simulink model "simulink_sim_V1"  (R2017a)
settings: Solver=FixedStepDiscrete  StartTime=0  StopTime=7  FixedStep=Ts  RelTol=1e-3  EnableMultiTasking=on
values from neighbouring files (symbols this model uses):
  Ts = 0.025    [ACADO_simulink.m]
  Xref = [0 0 0 0]    [ACADO_simulink.m]
undefined symbols (not defined in the file or in its folder): data, init, sigbuilder_block
settings Model: Creator=hirsch  LastModifiedBy=alvin
settings DataIOCC: LimitDataPoints=on  SaveFormat=Array  SignalLoggingSaveFormat=ModelDataLogs
settings OptimizationCC: ExpressionDepthLimit=2147483647  LifeSpan=inf
settings DebuggingCC: SolverPrmCheckMsg=warning  FcnCallInpInsideContextMsg=warning  StateNameClashWarn=warning  SFUnexpectedBacktrackingDiag=warning  SFNoUnconditionalDefaultTransitionDiag=warning  SFExecutionAtInitializationDiag=none
settings HardwareCC: ProdBitPerPointer=32  ProdBitPerSizeT=32  ProdBitPerPtrDiffT=32  ProdLargestAtomicFloat=None  ProdIntDivRoundTo=Undefined  ProdEndianess=Unspecified  ProdWordSize=32  ProdHWDeviceType=32-bit Generic
settings ModelReferenceCC: PropagateSignalLabelsOutOfModel=off
settings GRTTargetCC: TargetLangStandard=C89/C90 (ANSI)  GeneratePreprocessorConditionals=Disable all  CombineOutputUpdateFcns=off  GRTInterface=on
settings ConfigComp: CovMetricSettings=dw  CovHtmlReporting=on  CovSaveCumulativeToWorkspaceVar=on  CovSaveSingleToWorkspaceVar=on  CovExternalEMLEnable=off  CovSFcnEnable=off

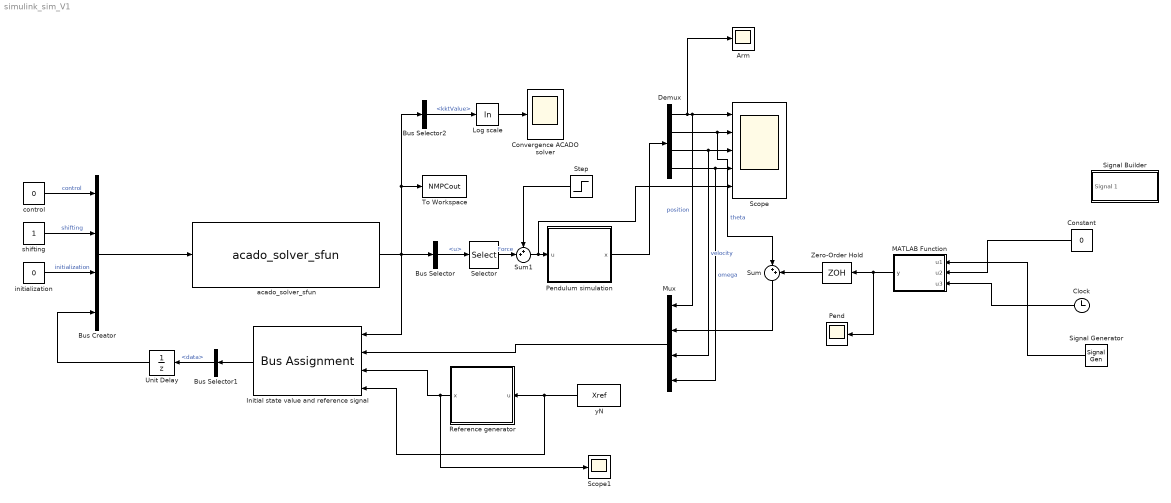
== system simulink_sim_V1 ==
  Arm : Scope
  Bus Creator : BusCreator  Inputs=4  OutDataTypeStr=Bus: ACADOinput
  Bus Selector : BusSelector  OutputSignals=data.u
  Bus Selector1 : BusSelector  OutputSignals=data
  Bus Selector2 : BusSelector  OutputSignals=kktValue
  Clock : Clock
  Constant : Constant  Value=0
  Convergence ACADO solver : Scope
  Demux : Demux
  Initial state value and reference signal : BusAssignment  AssignedSignals=data.x0,data.y,data.yN
  Log scale : Math  Operator=log  SaturateOnIntegerOverflow=on
  MATLAB Function : MATLAB Function  TreatAsAtomicUnit=on
  Mux : Mux
  Pend : Scope
  Pendulum simulation : Subsystem
      mask help: Simple system simulation.
      mask init:
      | % initialize state values
      mask Display: disp('System');
  Reference generator : Subsystem
      mask help: Simple system simulation.
      mask init:
      | % initialize state values
      mask Display: disp('System');
  Scope : Scope  NumInputPorts=5
  Scope1 : Scope
  Selector : Selector  InputPortWidth=80  IndexOptions=Starting index (dialog)  Indices=[1]  OutputSizes=1
  Signal Generator : SignalGenerator  Amplitude=0.1  Frequency=10  Units=rad/sec
  Signal Builder : Subsystem  Tag=STV Subsys  LoadFcn=sigbuilder_block('load');  StartFcn=sigbuilder_block('start');  StopFcn=sigbuilder_block('stop');  ClipboardFcn=sigbuilder_block('clipboard');  mask(Sigbuilder block){tuvar=[0:10]}
      mask help: Simulink:masks:SigbuilderBlock_MD
      mask init:
      | if ~strcmp(get_param(bdroot(gcbh),'SimulationStatus'),'stopped') tuvar = sigbuilder_block('maskInit'); end
      settings: CopyFcn=sigbuilder_block('copy');  DeleteFcn=sigbuilder_block('delete');  ModelCloseFcn=sigbuilder_block('modelClose');  PreSaveFcn=sigbuilder_block('preSave');  PauseFcn=sigbuilder_block('pause');  ContinueFcn=sigbuilder_block('continue');  NameChangeFcn=sigbuilder_block('namechange');  OpenFcn=sigbuilder_block('open',[94.5 0 580.5 448.5 ]);  CloseFcn=sigbuilder_block('close');
      mask Display: plot(0, 0, 100, 100,[2, 2, 32, 32, 2], [68, 8, 8, 68, 68],[32, 2], [38, 38], [32, 19, 2],[53, 60, 44], [32, 17, 17, 2],[16, 16, 31, 31]);txt = getActiveGroup(gcbh);text(2, 100, txt,'verticalAlignment', 'top');
  Step : Step  Time=4  After=0  SampleTime=0
  Sum : Sum  Inputs=|++
  Sum1 : Sum  Inputs=++|
  To Workspace : ToWorkspace  VariableName=NMPCout  SaveFormat=Timeseries  SampleTime=-1
  Unit Delay : UnitDelay  InitialCondition=init  SampleTime=Ts
  Zero-Order Hold : ZeroOrderHold  SampleTime=0.025
  acado_solver_sfun : S-Function  FunctionName=acado_solver_sfun  SFunctionDeploymentMode=off  EnableBusSupport=off  mask(Legacy Function){SFunctionSpec=acado_step(ACADOinput u1[1], ACADOoutput y1[1]), ShowSpec=on}
      mask prompts: ShowSpec "Display function specification"
      mask help:
      | This block allows you to call the legacy functions specified by the following Legacy Code Tool definition:
      | def.SFunctionName = 'acado_solver_sfun';
      | def.OutputFcnSpec = 'acado_step(ACADOinput u1[1], ACADOoutput y1[1])';
      | def.StartFcnSpec = 'acado_initialize( void )';
      | def.TerminateFcnSpec = 'acado_cleanup( void )';
      | def.HeaderFiles = {'acado_common.h', 'acado_solver_sfunction.h'};
      | def.SourceFiles = {'acado_solver.c', 'acado_integrator.c', 'acado_auxiliary_functions.c', 'acado_solver_sfunction.c', 'acado_qpoases_interface.cpp', 'qpoases/SRC/Bounds.cpp', 'qpoases/SRC/Constraints.cpp', 'qpoases/SRC/CyclingManager.cpp', 'qpoases/SRC/Indexlist.cpp', 'qpoases/SRC/MessageHandling.cpp', 'qpoases/SRC/QProblem.cpp', 'qpoases/SRC/QProblemB.cpp', 'qpoases/SRC/SubjectTo.cpp', 'qpoases/SRC/Utils.cpp', 'qpoases/SRC/EXTRAS/SolutionAnalysis.cpp'};
      | def.IncPaths = {'qpoases', 'qpoases/INCLUDE', 'qpoases/SRC'};
      | def.Options.language = 'C++';
      mask Help: <p>This block was generated automatically by the Legacy Code Tool. For detailed help on this tool, call<a href="matlab:legacy_code('help')"> legacy_code('help')</a>.</p>
      mask Callback ShowSpec:
      | if strcmp(get_param(gcbh, 'ShowSpec'), 'on')
      |   set_param(gcbh, 'MaskDisplay', sprintf('fprintf(''%s'');', get_param(gcbh, 'SFunctionSpec')));
      | else
      |   set_param(gcbh, 'MaskDisplay', sprintf('fprintf(''%s'');', get_param(gcbh, 'FunctionName')));
      | end
      mask Display: fprintf('acado_step(ACADOinput u1[1], ACADOoutput y1[1])');
  control : Constant  Value=0  OutDataTypeStr=int32
  initialization : Constant  Value=0  OutDataTypeStr=int32
  shifting : Constant  OutDataTypeStr=int32
  yN : Constant  Value=Xref  OutDataTypeStr=double
  wires:
  acado_solver_sfun/1 -> Bus Selector2/1, To Workspace/1, Initial state value and reference signal/1, Bus Selector/1
  Bus Selector/1 -> Selector/1  "<u>"
  shifting/1 -> Bus Creator/2  "shifting"
  control/1 -> Bus Creator/1  "control"
  initialization/1 -> Bus Creator/3  "initialization"
  Initial state value and reference signal/1 -> Bus Selector1/1
  Demux/1 -> Arm/1, Mux/1, Scope/1  "position"
  Demux/2 -> Sum/1, Scope/2  "theta"
  Demux/3 -> Mux/3, Scope/3  "velocity"
  Demux/4 -> Scope/4, Mux/4  "omega"
  Bus Creator/1 -> acado_solver_sfun/1
  Pendulum simulation/1(x) -> Demux/1
  Bus Selector1/1 -> Unit Delay/1  "<data>"
  Unit Delay/1 -> Bus Creator/4
  yN/1 -> Initial state value and reference signal/4, Reference generator/1(u)
  Reference generator/1(x) -> Scope1/1, Initial state value and reference signal/3
  Log scale/1 -> Convergence ACADO solver/1
  Bus Selector2/1 -> Log scale/1  "<kktValue>"
  Sum/1 -> Mux/2
  Mux/1 -> Initial state value and reference signal/2
  MATLAB Function/1(y) -> Pend/1, Zero-Order Hold/1
  Clock/1 -> MATLAB Function/3(u3)
  Selector/1 -> Sum1/2  "Force"
  Sum1/1 -> Scope/5, Pendulum simulation/1(u)
  Step/1 -> Sum1/1
  Zero-Order Hold/1 -> Sum/2
  Constant/1 -> MATLAB Function/2(u2)
  Signal Generator/1 -> MATLAB Function/1(u1)

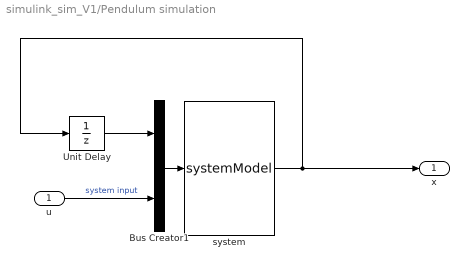
== system simulink_sim_V1/Pendulum simulation ==
  u : Inport
  Bus Creator1 : BusCreator  Inputs=2
  Unit Delay : UnitDelay  InitialCondition=init.x0  SampleTime=Ts
  system : S-Function  FunctionName=systemModel  SFunctionDeploymentMode=off  EnableBusSupport=off
  x : Outport
  wires:
  u/1 -> Bus Creator1/2  "system input"
  Bus Creator1/1 -> system/1
  system/1 -> x/1, Unit Delay/1
  Unit Delay/1 -> Bus Creator1/1

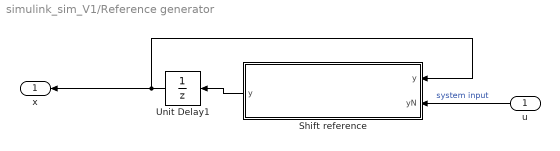
== system simulink_sim_V1/Reference generator ==
  u : Inport
  Shift reference : MATLAB Function  TreatAsAtomicUnit=on
  Unit Delay1 : UnitDelay  InitialCondition=init.y  SampleTime=Ts
  x : Outport
  wires:
  u/1 -> Shift reference/2(yN)  "system input"
  Shift reference/1(y) -> Unit Delay1/1
  Unit Delay1/1 -> x/1, Shift reference/1("y ")

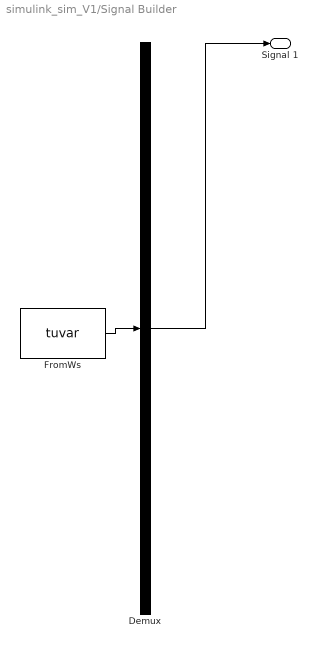
== system simulink_sim_V1/Signal Builder ==
  Demux : Demux  Tag=STV Demux  Outputs=1
  FromWs : FromWorkspace  Tag=STV FromWs  VariableName=tuvar  SampleTime=0
      SigBuilderData=|
      | common.afterFinalStr = 'Extrapolate'
      | common.sampleTime = 0
      | dataSet.timeRange = [0 10]
      | dataSet.name = 'Group 1'
      | sbobj.Groups.Name = 'Group 1'
      | sbobj.Groups.Signals.Name = 'Signal 1'
      | sbobj.Groups.Signals.XData = [0 4 4 4.1 4.1 10]
      | sbobj.Groups.Signals.YData = [0 0 0.3 0.3 0 0]
  Signal 1 : Outport  Tag=STV Outport
  wires:
  Demux/1 -> Signal 1/1
  FromWs/1 -> Demux/1

== matlab function simulink_sim_V1/MATLAB Function ==
  data: u1 input; y output; u2 input; u3 input
function y = fcn(u1,u2,u3)
%#codegen

if u3>4
    y = u1;
else
    y = u2;
end

== matlab function simulink_sim_V1/Reference generator/Shift reference ==
  data: y input; y output; yN input
function y = shift_reference(y, yN)

NX = 4;
NU = 1;

y = [y(NX+NU+1:end);yN;y(end-NU+1:end)];
